simulink model "base_reference"  (R2019a)
settings: Solver=ode23tb  StartTime=0.0  StopTime=60  RelTol=1e-3
model workspace (MAT data in the model file):
  A_mu = 10
  AxlIxx = 62.3745166667
  AxlM = 160
  B_reff = 8.386
  BattCapInit = 26
  BattChargeMax = 32.5
  BattChrgMax = -80000
  BattDischrgMax = 80000
  BattTempBp = [243.1 253.1 263.1 273.1 283.1 298.1 313.1]
  BrkPrsMax = 5000000
  CapLUTBp = [0 0.01 0.02 0.03 0.04 0.05 0.06 0.07 0.08 0.09 0.1 0.11 ... (101 elements, 1x101)]
  CapSOCBp = [0 0.2 0.4 0.6 0.8 1]
  ChrgLmt_bpt = [1 1 1 1 1 1 1 1 0.7 0.35 0]
  Cps = 2
  Cz = 5565.2246438
  CzWhlAxl = 11490.971257
  DCT_Param : struct (value not decoded)
  DLCXref = [0 6 7 14 33.5 34 42 50 60]
  DLCYref = [0 0 -4.5 -4 -3.75 1.5 0.5 0 0]
  D_reff = 0.25826
  DischrgLmt_bpt = [0 0.35 0.7 1 1 1 1 1 1 1 1]
  Downshift_Speeds = [9.5625 12.9375 16.3125 19.6875 23.0625 26.4375 29.8125 33.1875 36.5625 39.9375 43.3125 46.6875 ... (28 elements, 4x7)]
  EV_current = 200
  EV_motion = [20 4 0.8]
  EV_sf = 2000
  Em = [2.8 3.228 3.284 3.361 3.408 3.427 3.472 3.477 3.493 3.504 3.516 3.528 ... (101 elements, 1x101)]
  EngRevLim = 7000
  F0z = [2886 2907]
  F0zWhlAxl = 2907
  Fs = 0
  Fv = 0.0025
  Hmax = 0.25
  Jcomp = 0.0227
  Ki = 251.3274
  Kisa = 346.6583
  Kp_d = 0.47149
  Kp_q = 0.52125
  Ksa = 85.4316
  Ksf = 1996.2651
  Kz = 52451.0065793
  KzWhlAxl = 138031.612078
  Ld = 0.0003752
  Ldq = [0.0003752 0.0004148]
  Lq = 0.0004148
  Mechanical = [0.0227 0.0025 0]
  MotMapEff = 0
  MotSpd = [0 1000 2000 2728.370453 3000 4000 5000 6000 7000 8000 9000 10000]
  MotTrq = [280 280 280 280 254.6479089 190.9859317 152.7887454 127.3239545 109.1348181 95.49296586 84.88263632 76.39437268]
  NCyl = 6
  Ndiff = 7.94
  Np = 2
  Ns = 96
  P = 4
  Pedal_Positions = [0.1 0.4 0.5 0.9]
  PolePairs = 4
  Pstd = 101325
  RInt = [0.008846 0.006389 0.004364 0.002031 0.001443 0.0005603 0.001028 0.009319 0.006554 0.004101 0.002563 0.001825 ... (42 elements, 7x6)]
  Rair = 287
  RegenBrkCutOff = [0 1]
  RegenBrkSpd_bpt = [5 9]
  Rm = 0.15
  Rs = 0.2
  SOC_bpt = [0 10 20 30 40 50 60 70 80 90 100]
  SUS : struct (value not decoded)
  T_eff_bp = [0 20 40 60 80 100 120 140 160 180 200 220 ... (15 elements, 1x15)]
  T_max = 120
  T_mtpa = [0 13.3131834767 26.6278836885 39.9456159322 53.2678926341 66.5962219318 79.9321062746 93.277041051 106.632513247 120.000000141]
  Tc = 0.02
  Trans : struct (value not decoded)
  Tstd = 293.15
  Upshift_Speeds = [12.9375 16.3125 19.6875 33 26.4375 29.8125 33.1875 52.5 39.9375 43.3125 46.6875 77.25 ... (28 elements, 4x7)]
  VEH : struct (value not decoded)
  V_o = 16.7
  V_xlow = 1
  Vd = 0.00346
  WH : struct (value not decoded)
  a = 1.4
  alpha_max = 1.5
  alpha_min = -1.5
  b = 1.8
  ba = 3.4029
  c_zo = 209651
  disk_abore = 0.05
  dt3D = 0.05
  efficiency_table = [85 85 85 85 85 85 85 85 85 85 85 85 ... (180 elements, 12x15)]
  epsilon = 0.1
  f_air = [0 0 0 0 0 0 0 0 0 0 0 0 ... (256 elements, 16x16)]
  f_co = [0 0 0 0 0 0 0 0 0 0 0 0 ... (256 elements, 16x16)]
  f_co2 = [0 0 0 0 0 0 0 0 0 0 0 0 ... (256 elements, 16x16)]
  f_eff = [352.135682859 352.135682859 320.724378192 303.655312657 295.930136708 291.240087194 291.240271258 291.240312459 291.240275452 291.240198499 291.240100781 291.240018769 ... (256 elements, 16x16)]
  f_fuel = [0 0 0 0 0 0 0 0 0 0 0 0 ... (256 elements, 16x16)]
  f_hc = [0 0 0 0 0 0 0 0 0 0 0 0 ... (256 elements, 16x16)]
  f_nox = [0 0 0 0 0 0 0 0 0 0 0 0 ... (256 elements, 16x16)]
  f_pm = [0 0 0 0 0 0 0 0 0 0 0 0 ... (256 elements, 16x16)]
  f_susp_axl_bp = [1 2]
  f_susp_dz_bp = [-0.325022776267 -0.315022776267 -0.305022776267 -0.205022776267 -0.105022776267 -0.00502277626717 0.0949772237328 0.194977223733 0.204977223733 0.214977223733]
  f_susp_dzdot_bp = [-3 -0.3 -0.2 -0.1 0 0.1 0.2 0.3 3]
  f_susp_fmz = [-144070.391448 -93629.24037 -75929.1118915 -20630.5828179 -15385.48216 -10140.3815021 -4895.28084414 349.819813785 -31916.3973792 18437.6709544 -83996.1993354 -33555.0482577 ... (43920 elements, 10x9x61x2x4)]
  f_susp_geom = [0 0 0 0 0 0 0 0 0 0 0 0 ... (3660 elements, 10x61x2x3)]
  f_susp_strgdelta_bp = [-0.523598775598 -0.506145483078 -0.488692190558 -0.471238898038 -0.453785605519 -0.436332312999 -0.418879020479 -0.401425727959 -0.383972435439 -0.366519142919 -0.349065850399 -0.331612557879 ... (61 elements, 1x61)]
  f_tbrake = [0 76.8593923996 105.140482948 131.533638111 157.926793274 176.658631717 176.65727296 176.656856686 176.656879077 176.657093756 176.657404516 176.65772406 ... (256 elements, 16x16)]
  f_tbrake_n_bpt = [0 649.519052838 912.419621844 1175.32019085 1438.22075986 1701.12132886 1964.02189787 2226.92246687 2489.82303588 2752.72360489 3015.62417389 3278.5247429 ... (16 elements, 1x16)]
  f_tbrake_t_bpt = [0 34.6410161514 61.0341713143 87.4273264773 113.82048164 140.213636803 166.606791966 192.999947129 219.393102292 245.786257455 272.179412618 298.572567781 ... (16 elements, 1x16)]
  f_texh = [766.752464599 766.752464599 786.17542386 801.679939032 884.591982581 910.574397722 910.571871054 910.570774534 910.570601632 910.570821151 910.571247242 910.571639815 ... (256 elements, 16x16)]
  f_twc_eff_co = [0.17 0.25 0.45 0.99 0.99 0.99 0.99]
  f_twc_eff_hc = [0.21 0.375 0.75 0.98 0.98 0.98 0.98]
  f_twc_eff_lam = [0.909090909 0.944055944 0.979020979 1 1.013986014 1.048951049 1.083916084]
  f_twc_eff_nox = [0.98 0.98 0.98 0.97 0.05 0.02 0]
  h = 0.134
  id_mtpa = [0 -0.114523352646 -0.457989076459 -1.03008464374 -1.83029075221 -2.85788367342 -4.11193850568 -5.59133329791 -7.29475400168 -9.22070020138]
  idq0 = [0 0]
  idq_limits = [-9.220699542 166.993501392 167.247872355]
  iq_mtpa = [0 18.5827440345 37.1633719111 55.7397734896 74.3098506185 92.871523015 111.422734008 129.961456105 148.485696337 166.993501356]
  lambda_pm = 0.1194
  mechanical = [0.0227 0.0025 0]
  mu_kinetic = 0.35
  numWheel = 4
  num_pads = 2
  omega_init = 0
  path : struct (value not decoded)
  pio = 220000
  power_max = 80000
  q_Fcx = 0
  q_Fz2 = 15.4
  q_Fzy = 0
  q_reo = 0.9974
  q_sx1 = -0.007764
  q_sx10 = 0.2824
  q_sx11 = 5.349
  q_sx12 = 0
  q_sx13 = 0
  q_sx14 = 0
  q_sx2 = 1.1915
  q_sx3 = 0.013948
  q_sx4 = 4.912
  q_sx5 = 1.02
  q_sx6 = 22.83
  q_sx7 = 0.7104
  q_sx8 = -0.023393
  q_sx9 = 0.6581
  q_sy1 = 0.00702
  q_sy2 = 0
  q_sy3 = 0.001515
  q_sy4 = 8.514e-05
  q_sy5 = 0
  q_sy6 = 0
  q_sy7 = 0.9008
  q_sy8 = -0.4089
  q_v1 = 0.0007742
  q_v2 = 0.04667
  r_Bx1 = 12.531
  r_Bx2 = 9.532
  r_Bx3 = 0
  r_By1 = 10.615
  r_By2 = 7.705
  r_By3 = 3.433e-06
  r_By4 = 0
  r_Cx1 = 1.019
  r_Cy1 = 1.0585
  r_Ex1 = -0.4487
  r_Ex2 = -0.4726
  r_Ey1 = 0.3132
  r_Ey2 = 7.63e-06
  r_Hx1 = 0.0002374
  r_Hy1 = 0.011646
  r_Hy2 = 7.63e-06
  r_Vy1 = 0.05654
  r_Vy2 = 7.63e-06
  r_Vy3 = 0
  r_Vy4 = 99.9
  r_Vy5 = 2
  r_Vy6 = 15.814
  r_o = 0.3135
  theta_init = 0
  torque_max = 280
  vehWidth = 2
  w = 1
  w_eff_bp = [0 1000 2000 2728.370453 3000 4000 5000 6000 7000 8000 9000 10000]
values from neighbouring files (symbols this model uses):
  VEH =     [PassVeh14DOF.mat]    (also in model2.mat; model_workspace_reference.mat)
undefined symbols (not defined in the file or in its folder): Disabled, Right
libraries: simulink x8, vehdynlibtire x8, vehdynlibsuspension x7, autolibutils x6, vehdynlibscenariocommon x5, sim3dlib x4, autolibmappedmotor x4, autolibshared x2, sharedtransform x2, vehdynlibviscommon x2, vehdynlibdriver x1, vehdynlibsteering x1
(part 6 of 8)

== system base_reference/Passenger Vehicle/Subsystem6/Vehicle/Variant Subsystem/6DOF ==
  Suspension : Inport
  Wind : Inport  Port=2
  Bus Selector3 : BusSelector  OutputSignals=Veh.F,Veh.M
  Constant : Constant  Value=[0;0;0]
  Constant1 : Constant  Value=[0;0;0]
  Terminator{,1..5} (6 alike) : Terminator
  Vehicle Body 6DOF : vehdynlibeom/Vehicle Body 6DOF  extPos=on  extVel=on  extEuler=on  extRotRate=on  m=VEH.Mass  a=VEH.FrontAxlePositionfromCG  b=VEH.RearAxlePositionfromCG  d=0  h=VEH.HeightCG  Xe_o=[VEH.InitialLongPosition,VEH.InitialLatPosition,VEH.InitialVertPosition]  xbdot_o=[VEH.InitialLongVel,VEH.InitialLatVel,VEH.InitialVertVel]  eul_o=[VEH.InitialRollAngle,VEH.InitialPitchAngle,VEH.InitialYawAngle]  p_o=[VEH.InitialRollRate,VEH.InitialPitchRate,VEH.InitialYawRate]  Iveh=[VEH.RollMomentInertia 0 0; 0 VEH.PitchMomentInertia 0; 0 0 VEH.YawMomentInertia]  w=VEH.TrackWidth.*[1 1]  z1m=0  z1R=[-.25,.125,.15]  z1I=[1.4,-.2,.1;-.2,1.4,.1;.1,.1,2.25].*0  z2m=0  z2R=[1.4,0,.8]  z2I=[1.4,-.2,.1;-.2,1.4,.1;.1,.1,2.25].*0  z3m=0  z3R=[.75,-.5,.4]  z3I=[5,-.1,-2;-2,9,.1;-.1,.1,6].*0  z4m=0  z4R=[.75,.5,.4]  z4I=[5,-.1,-2;-2,9,.1;-.1,.1,6].*0  z5m=0  z5R=[1.25,-.5,.4]  z5I=[5,-.1,-2;-2,9,.1;-.1,.1,6].*0  z6m=0  z6R=[1.25,-.5,.4]  z6I=[5,-.1,-2;-2,9,.1;-.1,.1,6].*0  z7m=0  z7R=[2,0,.25]  z7I=[1.4,-.2,.1;-.2,1.4,.1;.1,.1,2.25].*0  Af=VEH.FrontalArea  Cd=.3  Cl=.1  Cpm=.1  beta_w=[0:0.01:0.3]  Cs=[0:0.03:0.9]  Cym=[0:0.01:0.3]  Pabs=101325  extTamb=off  Tair=273  g=9.81  xdot_tol=.1  longOff=0  latOff=0  vertOff=0.0112  wrapAng=on  aMode=2
      settings: SourceProductName=Vehicle Dynamics Blockset  SourceProductBaseCode=VE
  VehFdbk : Outport
  wires:
  Bus Selector3/2 -> Vehicle Body 6DOF/2  "<M>"
  Bus Selector3/1 -> Vehicle Body 6DOF/1  "<F>"
  Wind/1 -> Vehicle Body 6DOF/5
  Constant/1 -> Vehicle Body 6DOF/3
  Suspension/1 -> Bus Selector3/1
  Vehicle Body 6DOF/1 -> VehFdbk/1  "VehFdbk"
  Constant1/1 -> Vehicle Body 6DOF/4
  Vehicle Body 6DOF/2 -> Terminator/1
  Vehicle Body 6DOF/3 -> Terminator1/1
  Vehicle Body 6DOF/4 -> Terminator2/1
  Vehicle Body 6DOF/5 -> Terminator3/1
  Vehicle Body 6DOF/6 -> Terminator4/1
  Vehicle Body 6DOF/7 -> Terminator5/1

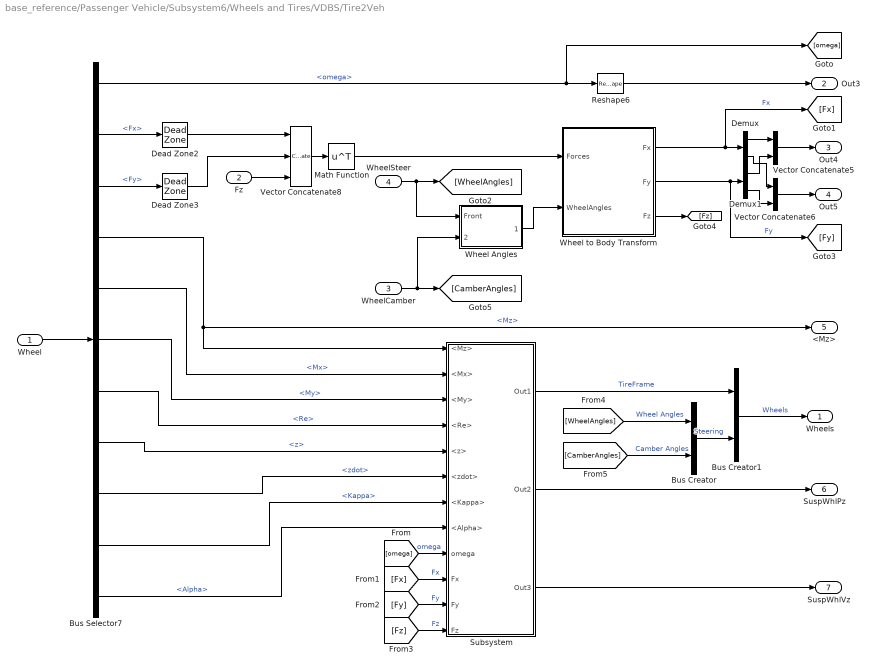
== system base_reference/Passenger Vehicle/Subsystem6/Wheels and Tires/VDBS/Tire2Veh ==
  Wheel : Inport
  Fz : Inport  Port=2
  WheelCamber : Inport  Port=3
  WheelSteer : Inport  Port=4
  Bus Creator : BusCreator  Inputs=2
  Bus Creator1 : BusCreator  Inputs=2
  Bus Selector7 : BusSelector  OutputSignals=omega,Fx,Fy,Mz,Mx,My,Re,z,zdot,Kappa,Alpha
  Dead Zone2 : DeadZone  LowerValue=-5  UpperValue=5  ZeroCross=off  SaturateOnIntegerOverflow=on
  Dead Zone3 : DeadZone  LowerValue=-10  UpperValue=10  ZeroCross=off  SaturateOnIntegerOverflow=on
  Demux : Demux  Outputs=[2,2]
  Demux1 : Demux  Outputs=[2,2]
  Math Function : Math  Operator=transpose  SaturateOnIntegerOverflow=on
  Reshape6 : Reshape  OutputDimensionality=Customize  OutputDimensions=[2,2]
  Subsystem : Subsystem
  Vector Concatenate5 : Concatenate  Mode=Multidimensional array  ConcatenateDimension=2
  Vector Concatenate6 : Concatenate  Mode=Multidimensional array  ConcatenateDimension=2
  Vector Concatenate8 : Concatenate  NumInputs=3  Mode=Multidimensional array  ConcatenateDimension=2
  Wheel Angles : Subsystem
  Wheel to Body Transform : Subsystem
  Wheels : Outport
  Out3 : Outport  Port=2
  Out4 : Outport  Port=3
  Out5 : Outport  Port=4
  <Mz> : Outport  Port=5
  SuspWhlPz : Outport  Port=6
  SuspWhlVz : Outport  Port=7
  wires:
  Fz/1 -> Vector Concatenate8/3
  Vector Concatenate6/1 -> Out5/1
  Vector Concatenate8/1 -> Math Function/1
  Demux/2 -> Vector Concatenate6/1
  Demux1/2 -> Vector Concatenate6/2
  Demux/1 -> Vector Concatenate5/1
  Math Function/1 -> Wheel to Body Transform/1(Forces)
  Dead Zone3/1 -> Vector Concatenate8/2
  Bus Selector7/2 -> Dead Zone2/1  "<Fx>"
  Dead Zone2/1 -> Vector Concatenate8/1
  Wheel to Body Transform/1(Fx) -> [Fx], Demux/1  "Fx"
  Vector Concatenate5/1 -> Out4/1
  Wheel/1 -> Bus Selector7/1
  Reshape6/1 -> Out3/1
  Demux1/1 -> Vector Concatenate5/2
  Wheel to Body Transform/2(Fy) -> Demux1/1, [Fy]  "Fy"
  Wheel Angles/1(Vehicle) -> Wheel to Body Transform/2(WheelAngles)
  Bus Selector7/1 -> [omega], Reshape6/1  "<omega>"
  WheelSteer/1 -> Wheel Angles/1(Front), [WheelAngles]
  Bus Selector7/4 -> <Mz>/1, Subsystem/1(<Mz>)  "<Mz>"
  Wheel to Body Transform/3(Fz) -> [Fz]
  WheelCamber/1 -> Wheel Angles/2(Camber), [CamberAngles]
  Bus Selector7/3 -> Dead Zone3/1  "<Fy>"
  Bus Selector7/5 -> Subsystem/2(<Mx>)  "<Mx>"
  Bus Selector7/6 -> Subsystem/3(<My>)  "<My>"
  Bus Selector7/7 -> Subsystem/4(<Re>)  "<Re>"
  [omega] -> Subsystem/9(omega)  "omega"
  [Fx] -> Subsystem/10(Fx)  "Fx"
  Bus Selector7/8 -> Subsystem/5(<z>)  "<z>"
  [Fy] -> Subsystem/11(Fy)  "Fy"
  [Fz] -> Subsystem/12(Fz)  "Fz"
  Bus Selector7/9 -> Subsystem/6(<zdot>)  "<zdot>"
  Bus Selector7/10 -> Subsystem/7(<Kappa>)  "<Kappa>"
  Subsystem/2(Out2) -> SuspWhlPz/1
  Subsystem/3(Out3) -> SuspWhlVz/1
  [WheelAngles] -> Bus Creator/1  "Wheel Angles"
  Bus Creator1/1 -> Wheels/1  "Wheels"
  Subsystem/1(Out1) -> Bus Creator1/1  "TireFrame"
  [CamberAngles] -> Bus Creator/2  "Camber Angles"
  Bus Creator/1 -> Bus Creator1/2  "Steering"
  Bus Selector7/11 -> Subsystem/8(<Alpha>)  "<Alpha>"

== system base_reference/Passenger Vehicle/Subsystem6/Wheels and Tires/VDBS/Tires ==
  "DriveTorque " : Inport
  "Brake Pressure " : Inport  Port=2
  "r " : Inport  Port=3
  "Vx " : Inport  Port=4
  "Vy " : Inport  Port=5
  "Camber " : Inport  Port=6
  "Press " : Inport  Port=7
  "lambda " : Inport  Port=8
  "Gnd " : Inport  Port=9
  "FzSusp " : Inport  Port=10
  Fiala Tires : Subsystem  VariantControl=1
  MF Tires : Subsystem  VariantControl=0
  " Wheels" : Outport

== system base_reference/Passenger Vehicle/Subsystem6/Wheels and Tires/VDBS/Veh2Tire ==
  r : Inport
  Axle : Inport  Port=2
  Brake : Inport  Port=3
  VehVel : Inport  Port=4
  WheelSteer : Inport  Port=5
  WheelCamber : Inport  Port=6
  Demux4 : Demux
  Gain4 : Gain  Gain=[1;-1;1;-1]*0+1
  Mux1 : Mux
  Reshape3 : Reshape
  Reshape4 : Reshape
  Unary Minus : UnaryMinus
  Wheel Angles : Subsystem
  Wheel to Body Transform : Subsystem
  T : Outport  Unit=N*m
  P : Outport  Port=2  Unit=Pa
  psidot : Outport  Port=3  Unit=rad/s
  xdotAxle : Outport  Port=4  Unit=m/s
  ydotAxle : Outport  Port=5  Unit=m/s
  zdotAxle : Outport  Port=6  Unit=m/s
  wires:
  Demux4/1 -> Mux1/1
  Brake/1 -> Reshape3/1
  Demux4/4 -> Mux1/4
  Axle/1 -> Reshape4/1
  Wheel to Body Transform/1(xdotWheel) -> xdotAxle/1  "Vx"
  Demux4/2 -> Mux1/2
  Wheel to Body Transform/2(ydotWheel) -> ydotAxle/1  "Vy"
  WheelSteer/1 -> Wheel Angles/1(steer)
  Mux1/1 -> P/1
  r/1 -> Unary Minus/1
  Demux4/3 -> Mux1/3
  Reshape3/1 -> Demux4/1
  Gain4/1 -> T/1
  Reshape4/1 -> Gain4/1
  VehVel/1 -> Wheel to Body Transform/1(VelVeh)
  Wheel to Body Transform/3(zdotWheel) -> zdotAxle/1  "Vz"
  WheelCamber/1 -> Wheel Angles/2(camber)
  Unary Minus/1 -> psidot/1
  Wheel Angles/1(Vehicle) -> Wheel to Body Transform/2(WheelAngles)

== system base_reference/Passenger Vehicle/Subsystem6/Wheels and Tires/VDBS/scale factors with friction ==
  lamda_mu_x : Inport
  lamda_mu_y : Inport  Port=2
  Reshape : Reshape  OutputDimensionality=Row vector (2-D)  OutputDimensions=[1,numWheels]
  Reshape1 : Reshape  OutputDimensionality=Row vector (2-D)  OutputDimensions=[1,numWheels]
  Signal Specification : SignalSpecification  Unit=1
  Signal Specification1 : SignalSpecification  Unit=1
  Vector Concatenate : Concatenate  NumInputs=4  Mode=Multidimensional array
  ones1 : Constant  Value=[ones(24,numWheels)]  VectorParams1D=off
  ones2 : Constant  Value=ones(1,numWheels)  VectorParams1D=off
  lambdas : Outport  Unit=1
  wires:
  Reshape1/1 -> Vector Concatenate/3
  Reshape/1 -> Vector Concatenate/2
  lamda_mu_y/1 -> Reshape1/1
  lamda_mu_x/1 -> Reshape/1
  ones1/1 -> Signal Specification1/1
  ones2/1 -> Signal Specification/1
  Vector Concatenate/1 -> lambdas/1
  Signal Specification/1 -> Vector Concatenate/1
  Signal Specification1/1 -> Vector Concatenate/4

== system base_reference/Reference Generator/3D Engine/3D Engine/Scale/PartConcatenation ==
  BodyX : Inport
  BodyY : Inport  Port=2
  BodyZ : Inport  Port=3
  WheelFrontLeftX : Inport  Port=4
  WheelFrontLeftY : Inport  Port=5
  WheelFrontLeftZ : Inport  Port=6
  WheelFrontRightX : Inport  Port=7
  WheelFrontRightY : Inport  Port=8
  WheelFrontRightZ : Inport  Port=9
  WheelRearLeftX : Inport  Port=10
  WheelRearLeftY : Inport  Port=11
  WheelRearLeftZ : Inport  Port=12
  WheelRearRightX : Inport  Port=13
  WheelRearRightY : Inport  Port=14
  WheelRearRightZ : Inport  Port=15
  AllParts : Concatenate  NumInputs=5  Mode=Multidimensional array
  Body : Concatenate  NumInputs=3  Mode=Multidimensional array  ConcatenateDimension=2
  WheelFrontLeft : Concatenate  NumInputs=3  Mode=Multidimensional array  ConcatenateDimension=2
  WheelFrontRight : Concatenate  NumInputs=3  Mode=Multidimensional array  ConcatenateDimension=2
  WheelRearLeft : Concatenate  NumInputs=3  Mode=Multidimensional array  ConcatenateDimension=2
  WheelRearRight : Concatenate  NumInputs=3  Mode=Multidimensional array  ConcatenateDimension=2
  ConcatOut : Outport
  wires:
  BodyX/1 -> Body/1
  BodyZ/1 -> Body/3
  WheelFrontLeftX/1 -> WheelFrontLeft/1
  WheelFrontLeftZ/1 -> WheelFrontLeft/3
  WheelFrontLeftY/1 -> WheelFrontLeft/2
  BodyY/1 -> Body/2
  WheelFrontLeft/1 -> AllParts/2
  WheelRearRightX/1 -> WheelRearRight/1
  Body/1 -> AllParts/1
  WheelRearLeft/1 -> AllParts/4
  WheelFrontRight/1 -> AllParts/3
  WheelRearRightZ/1 -> WheelRearRight/3
  WheelFrontRightY/1 -> WheelFrontRight/2
  WheelFrontRightX/1 -> WheelFrontRight/1
  WheelRearRightY/1 -> WheelRearRight/2
  WheelRearLeftZ/1 -> WheelRearLeft/3
  AllParts/1 -> ConcatOut/1
  WheelRearLeftY/1 -> WheelRearLeft/2
  WheelRearRight/1 -> AllParts/5
  WheelRearLeftX/1 -> WheelRearLeft/1
  WheelFrontRightZ/1 -> WheelFrontRight/3

== system base_reference/Passenger Vehicle/Subsystem6/Wheels and Tires/VDBS/Tire2Veh/Subsystem ==
  <Mz> : Inport
  <Mx> : Inport  Port=2
  <My> : Inport  Port=3
  <Re> : Inport  Port=4
  <z> : Inport  Port=5
  <zdot> : Inport  Port=6
  <Kappa> : Inport  Port=7
  <Alpha> : Inport  Port=8
  omega : Inport  Port=9
  Fx : Inport  Port=10
  Fy : Inport  Port=11
  Fz : Inport  Port=12
  Bus Creator : BusCreator  Inputs=12
  Reshape : Reshape  OutputDimensionality=Row vector (2-D)
  Reshape1 : Reshape  OutputDimensionality=Row vector (2-D)
  Unary Minus1 : UnaryMinus
  Unary Minus2 : UnaryMinus
  Out1 : Outport
  Out2 : Outport  Port=2
  Out3 : Outport  Port=3
  wires:
  <Re>/1 -> Bus Creator/8
  Unary Minus1/1 -> Reshape/1, Bus Creator/9  "z"
  Fz/1 -> Bus Creator/4
  <zdot>/1 -> Unary Minus2/1
  <Mz>/1 -> Bus Creator/7
  Unary Minus2/1 -> Reshape1/1, Bus Creator/10  "zdot"
  <z>/1 -> Unary Minus1/1
  Bus Creator/1 -> Out1/1
  Fy/1 -> Bus Creator/3
  omega/1 -> Bus Creator/1
  Fx/1 -> Bus Creator/2
  Reshape1/1 -> Out3/1
  <Kappa>/1 -> Bus Creator/11
  Reshape/1 -> Out2/1
  <Mx>/1 -> Bus Creator/5
  <My>/1 -> Bus Creator/6
  <Alpha>/1 -> Bus Creator/12

== system base_reference/Passenger Vehicle/Subsystem6/Wheels and Tires/VDBS/Tire2Veh/Wheel Angles ==
  Front : Inport
  Camber : Inport  Port=2
  Add1 : Sum
  Add2 : Sum
  Constant1 : Constant  Value=pi
  Constant2 : Constant  Value=[pi;0;pi;0].*0+[0;pi;0;pi].*.0
  Constant3 : Constant  Value=ones(1,4).*0
  Reshape : Reshape  OutputDimensionality=Row vector (2-D)
  Reshape1 : Reshape  OutputDimensionality=Row vector (2-D)
  Reshape2 : Reshape  OutputDimensionality=Row vector (2-D)
  Vector Concatenate3 : Concatenate  NumInputs=3  Mode=Multidimensional array
  Vehicle : Outport
  wires:
  Reshape/1 -> Vector Concatenate3/3
  Reshape2/1 -> Vector Concatenate3/2
  Vector Concatenate3/1 -> Vehicle/1
  Constant2/1 -> Add1/2
  Front/1 -> Add1/1
  Reshape1/1 -> Vector Concatenate3/1
  Constant3/1 -> Reshape2/1
  Add1/1 -> Reshape/1
  Camber/1 -> Add2/1
  Add2/1 -> Reshape1/1
  Constant1/1 -> Add2/2

== system base_reference/Passenger Vehicle/Subsystem6/Wheels and Tires/VDBS/Tire2Veh/Wheel to Body Transform ==
  Forces : Inport  Partition=on  PartitionDimension=2  PartitionWidth=1  PartitionOffset=0
  WheelAngles : Inport  Port=2  Partition=on  PartitionDimension=2  PartitionWidth=1  PartitionOffset=0
  Demux1 : Demux  Outputs=3
  Divide1 : Product  Inputs=**  Multiplication=Matrix(*)
  For Each : ForEach  DisableCoverage=on  IndexMode=One-based
  Rotation Angles to Direction Cosine Matrix : sharedtransform/Rotation Angles to Direction Cosine Matrix  rotationOrder=ZYX  aMode=2
      settings: SourceProductBaseCode=AE
  Selector : Selector  InputPortWidth=3  IndexOptions=Index vector (dialog)  Indices=[3 2 1]  OutputSizes=1
  Fx : Outport  ConcatenationDimension=1
  Fy : Outport  Port=2  ConcatenationDimension=1
  Fz : Outport  Port=3  ConcatenationDimension=1
  wires:
  Divide1/1 -> Demux1/1
  Demux1/1 -> Fx/1
  Demux1/2 -> Fy/1
  Demux1/3 -> Fz/1
  Rotation Angles to Direction Cosine Matrix/1 -> Divide1/1
  Forces/1 -> Divide1/2
  WheelAngles/1 -> Selector/1
  Selector/1 -> Rotation Angles to Direction Cosine Matrix/1
